simulink model "model_proces_etapa1"  (R2020a)
settings: Solver=VariableStepAuto  StartTime=0.0  StopTime=500  RelTol=1e-3
settings Model: Creator=user  LastModifiedBy=user

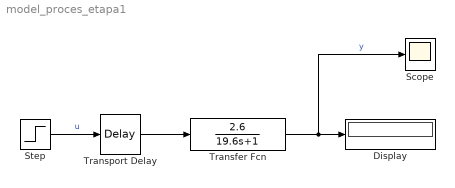
== system model_proces_etapa1 ==
  Display : Display
  Scope : Scope
  Step : Step  SampleTime=0
  Transfer Fcn : TransferFcn  Numerator=[2.6]  Denominator=[19.6 1]
  Transport Delay : TransportDelay  DelayTime=5
  wires:
  Step/1 -> Transport Delay/1  "u"
  Transfer Fcn/1 -> Scope/1, Display/1  "y"
  Transport Delay/1 -> Transfer Fcn/1
